simulink model "Update_E_Bike_model_without_controller"  (R2019b)
settings: Solver=VariableStepAuto  StartTime=0.0  StopTime=1000  RelTol=1e-3
InitFcn:
  | Rho_air= 1.225;
  | C_d=0.9;
  | A_d= 0.4;
  | Static_Friction_Coefficient =0.0015;
  | Dynamic_Friction_Coefficient= 0.0015;
  | Cyclist_weight=85;
  | Vehicle_mass = 5;
  | g = 9.81;
  | Wheel_Inertia = 0.45;
  | Bb=0.2;
  | Wheel_Radius = 0.3;
  | F_Rider = 100;
  | Brake_Pressure = 0;
  | Crank_Length = 0.150;
  | Angle_of_crank = [0:1:360;0:1:360;]';
  | Number_of_brake_pad = 2;
  | Coefficient_of_Brake_friction = 0.9;
  | Effective_Radius_of_Disc = 0.16;
  | Outer_Radius_of_Brake = 0.18;
  | Inner_Radius_of_Brake = 0.14;
  | Disc_Mass=0;
  | Heat_capacity=0;
  | Surface_Temp=0;
  | Ambient_Temp=0;
  | Thermal_Conductivity=1;
  | 
  | Motor_torque_constant = 1.41; % NM/A
  | Kb = (1/(190*2*pi/60)); %or  V/Wm (wm in rps) volt/rps
  | Jm =11.6 *10^-7; %kgm^2
  | Bm = ((Motor_torque_constant)*(20*10^-3)/(9080*2*pi/60));
  | Motor_resistance =250*10^-3; %ohm
  | L = .82*10^-3;% H(henry)
  | alpha_Conductor =0.0040;
  | Ref_Temp = 25;
  | Alpha_Magnet = -0.0020;
  | 
  | Current =2; %A
  | Internal_Resistance = 95*10^-3; %ohm
  | capacity = 14.5 ; %Ah
  | SOC_initial = 100;
  | Polarization_Resistance = 95*10^-3;
  | Polarization_Capacitance = 1*10^-7;
  | bp.SOC0_pct=00
undefined symbols (not defined in the file or in its folder): sigbuilder_block
(part 1 of 3)
settings Model: Creator=Avmash  LastModifiedBy=Avmash
settings DataIOCC: ReturnWorkspaceOutputs=off
settings DebuggingCC: AlgebraicLoopMsg=none  ArithmeticOperatorsInVariantConditions=warning
settings SFSimCC: SimUseLocalCustomCode=off  CustomCodeUndefinedFunction=UseInterfaceOnly
settings RTWCC: RTWUseLocalCustomCode=off

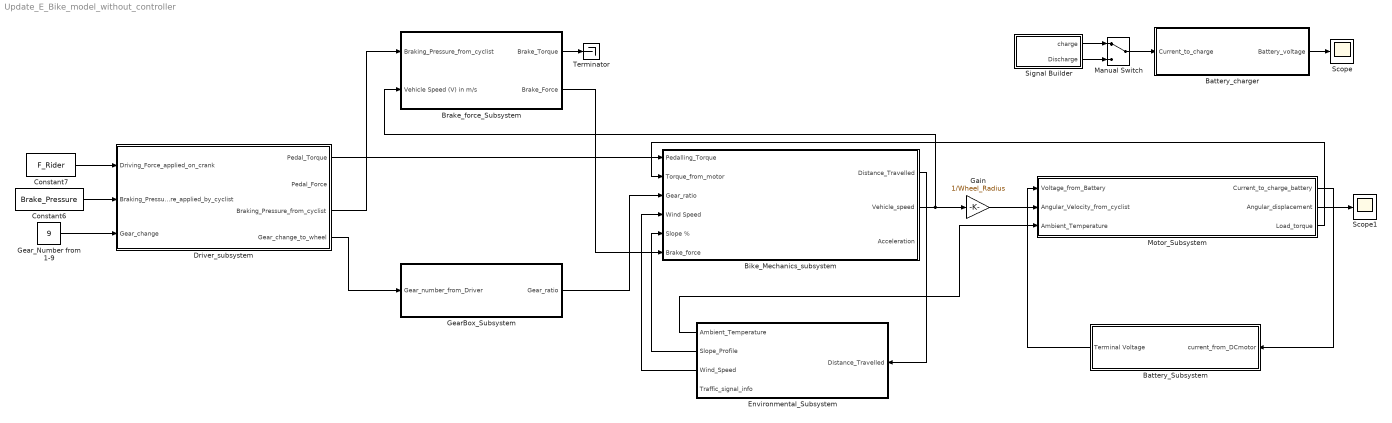
== system Update_E_Bike_model_without_controller ==
  Battery_Subsystem : Subsystem
  Battery_charger : Subsystem
  Bike_Mechanics_subsystem : Subsystem
  Brake_force_Subsystem : Subsystem
  Constant6 : Constant  Value=Brake_Pressure
  Constant7 : Constant  Value=F_Rider
  Driver_subsystem : Subsystem
  Environmental_Subsystem : Subsystem
  Gain : Gain  Gain=1/Wheel_Radius
  GearBox_Subsystem : Subsystem
  Gear_Number from 1-9 : Constant  Value=9
  Manual Switch : ManualSwitch
  Motor_Subsystem : Subsystem
  Scope : Scope
  Scope1 : Scope
  Signal Builder : Subsystem  Tag=STV Subsys  LoadFcn=sigbuilder_block('load');  StartFcn=sigbuilder_block('start');  StopFcn=sigbuilder_block('stop');  ClipboardFcn=sigbuilder_block('clipboard');  mask(Sigbuilder block){tuvar=[0:10]}
      mask help: Simulink:masks:SigbuilderBlock_MD
      mask init:
      | if ~strcmp(get_param(bdroot(gcbh),'SimulationStatus'),'stopped') tuvar = sigbuilder_block('maskInit'); end
      settings: CopyFcn=sigbuilder_block('copy');  DeleteFcn=sigbuilder_block('delete');  ModelCloseFcn=sigbuilder_block('modelClose');  PreSaveFcn=sigbuilder_block('preSave');  PauseFcn=sigbuilder_block('pause');  ContinueFcn=sigbuilder_block('continue');  NameChangeFcn=sigbuilder_block('namechange');  OpenFcn=sigbuilder_block('open',[6 30 1012.5 447.75 ]);  CloseFcn=sigbuilder_block('close');
      mask Display: plot(0, 0, 100, 100,[2, 2, 32, 32, 2], [68, 8, 8, 68, 68],[32, 2], [38, 38], [32, 19, 2],[53, 60, 44], [32, 17, 17, 2],[16, 16, 31, 31]);txt = getActiveGroup(gcbh);text(2, 100, txt,'verticalAlignment', 'top');
  Terminator : Terminator
  wires:
  Constant6/1 -> Driver_subsystem/2(Braking_Pressure_applied_by_cyclist)
  Gear_Number from 1-9/1 -> Driver_subsystem/3(Gear_change)
  Constant7/1 -> Driver_subsystem/1(Driving_Force_applied_on_crank)
  Brake_force_Subsystem/2(Brake_Force) -> Bike_Mechanics_subsystem/6("Brake_force ")
  Brake_force_Subsystem/1(Brake_Torque) -> Terminator/1
  Driver_subsystem/3(Braking_Pressure_from_cyclist) -> Brake_force_Subsystem/1(Braking_Pressure_from_cyclist)
  Driver_subsystem/1(Pedal_Torque) -> Bike_Mechanics_subsystem/1(Pedalling_Torque)
  Driver_subsystem/4(Gear_change_to_wheel) -> GearBox_Subsystem/1(Gear_number_from_Driver)
  GearBox_Subsystem/1(Gear_ratio) -> Bike_Mechanics_subsystem/3(Gear_ratio)
  Environmental_Subsystem/2(Slope_Profile) -> Bike_Mechanics_subsystem/5(Slope %)
  Environmental_Subsystem/3(Wind_Speed) -> Bike_Mechanics_subsystem/4(Wind Speed)
  Bike_Mechanics_subsystem/1(Distance_Travelled) -> Environmental_Subsystem/1(Distance_Travelled)
  Manual Switch/1 -> Battery_charger/1(Current_to_charge)
  Battery_charger/1(Battery_voltage) -> Scope/1
  Signal Builder/1(charge) -> Manual Switch/1
  Signal Builder/2(Discharge) -> Manual Switch/2
  Battery_Subsystem/1(Terminal Voltage) -> Motor_Subsystem/1(Voltage_from_Battery)
  Environmental_Subsystem/1(Ambient_Temperature) -> Motor_Subsystem/3(Ambient_Temperature)
  Motor_Subsystem/1(Current_to_charge_battery) -> Battery_Subsystem/1(current_from_DCmotor)
  Gain/1 -> Motor_Subsystem/2(Angular_Velocity_from_cyclist)
  Bike_Mechanics_subsystem/2(Vehicle_speed) -> Gain/1, Brake_force_Subsystem/2(Vehicle Speed (V) in m/s)
  Motor_Subsystem/3(Load_torque) -> Bike_Mechanics_subsystem/2(Torque_from_motor)
  Motor_Subsystem/2(Angular_displacement) -> Scope1/1

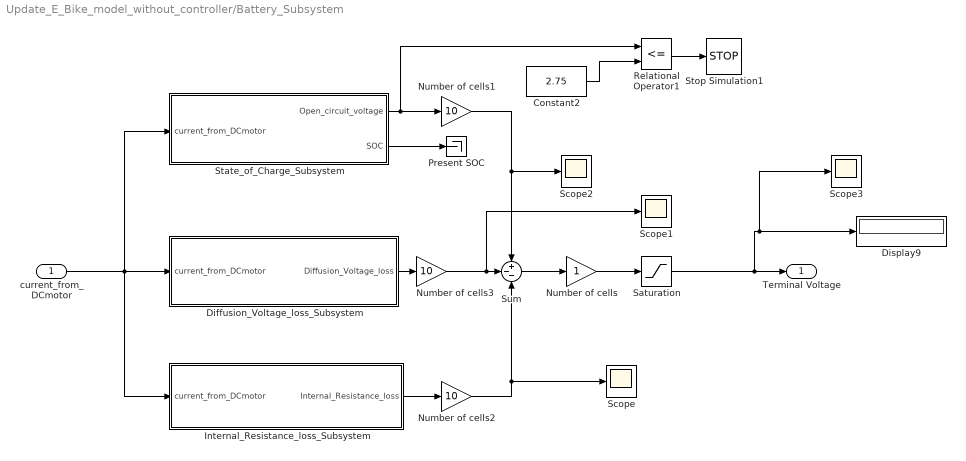
== system Update_E_Bike_model_without_controller/Battery_Subsystem ==
  current_from_DCmotor : Inport
  Constant2 : Constant  Value=2.75
  Diffusion_Voltage_loss_Subsystem : Subsystem
  Display9 : Display
  Internal_Resistance_loss_Subsystem : Subsystem
  Number of cells : Gain
  Number of cells1 : Gain  Gain=10
  Number of cells2 : Gain  Gain=10
  Number of cells3 : Gain  Gain=10
  Present SOC : Terminator
  Relational Operator1 : RelationalOperator  Operator=<=  OutDataTypeStr=boolean  RndMeth=Simplest
  Saturation : Saturate  UpperLimit=inf  LowerLimit=0
  Scope{,1..3} (4 alike) : Scope
  "State_of_Charge_Subsystem " : Subsystem
  Stop Simulation1 : Stop
  Sum : Sum  Inputs=+--
  Terminal Voltage : Outport  VectorParamsAs1DForOutWhenUnconnected=off
  wires:
  current_from_DCmotor/1 -> Internal_Resistance_loss_Subsystem/1(current_from_DCmotor), "State_of_Charge_Subsystem "/1(current_from_DCmotor), Diffusion_Voltage_loss_Subsystem/1(current_from_DCmotor)
  Sum/1 -> Number of cells/1
  "State_of_Charge_Subsystem "/2(SOC) -> Present SOC/1
  Internal_Resistance_loss_Subsystem/1(Internal_Resistance_loss) -> Number of cells2/1
  Number of cells/1 -> Saturation/1
  Diffusion_Voltage_loss_Subsystem/1(Diffusion_Voltage_loss) -> Number of cells3/1
  Saturation/1 -> Terminal Voltage/1, Scope3/1, Display9/1
  Relational Operator1/1 -> Stop Simulation1/1
  Constant2/1 -> Relational Operator1/2
  "State_of_Charge_Subsystem "/1(Open_circuit_voltage) -> Number of cells1/1, Relational Operator1/1
  Number of cells2/1 -> Scope/1, Sum/3
  Number of cells3/1 -> Scope1/1, Sum/2
  Number of cells1/1 -> Scope2/1, Sum/1

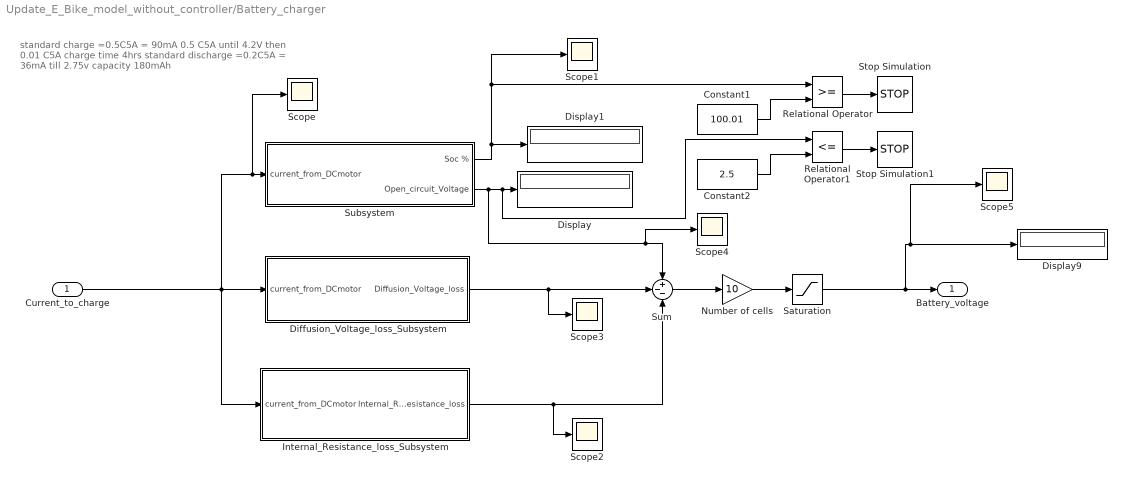
== system Update_E_Bike_model_without_controller/Battery_charger ==
  note: standard charge =0.5C5A = 90mA
      | 0.5 C5A until 4.2V then 0.01 C5A charge time 4hrs
      |
      | standard discharge =0.2C5A = 36mA till 2.75v
      |
      | capacity 180mAh
  Current_to_charge : Inport
  Constant1 : Constant  Value=100.01
  Constant2 : Constant  Value=2.5
  Diffusion_Voltage_loss_Subsystem : Subsystem
  Display : Display
  Display1 : Display
  Display9 : Display
  Internal_Resistance_loss_Subsystem : Subsystem
  Number of cells : Gain  Gain=10
  Relational Operator : RelationalOperator  OutDataTypeStr=boolean  RndMeth=Simplest
  Relational Operator1 : RelationalOperator  Operator=<=  OutDataTypeStr=boolean  RndMeth=Simplest
  Saturation : Saturate  UpperLimit=inf  LowerLimit=0
  Scope{,1..5} (6 alike) : Scope
  Stop Simulation : Stop
  Stop Simulation1 : Stop
  Subsystem : Subsystem
  Sum : Sum  Inputs=+--
  Battery_voltage : Outport  VectorParamsAs1DForOutWhenUnconnected=off
  wires:
  Saturation/1 -> Battery_voltage/1, Scope5/1, Display9/1
  Constant2/1 -> Relational Operator1/2
  Subsystem/2(Open_circuit_Voltage) -> Relational Operator1/1, Display/1, Scope4/1, Sum/1
  Diffusion_Voltage_loss_Subsystem/1(Diffusion_Voltage_loss) -> Sum/2, Scope3/1
  Current_to_charge/1 -> Scope/1, Subsystem/1(current_from_DCmotor), Internal_Resistance_loss_Subsystem/1(current_from_DCmotor), Diffusion_Voltage_loss_Subsystem/1(current_from_DCmotor)
  Sum/1 -> Number of cells/1
  Subsystem/1(Soc %) -> Relational Operator/1, Scope1/1, Display1/1
  Internal_Resistance_loss_Subsystem/1(Internal_Resistance_loss) -> Sum/3, Scope2/1
  Number of cells/1 -> Saturation/1
  Relational Operator/1 -> Stop Simulation/1
  Constant1/1 -> Relational Operator/2
  Relational Operator1/1 -> Stop Simulation1/1

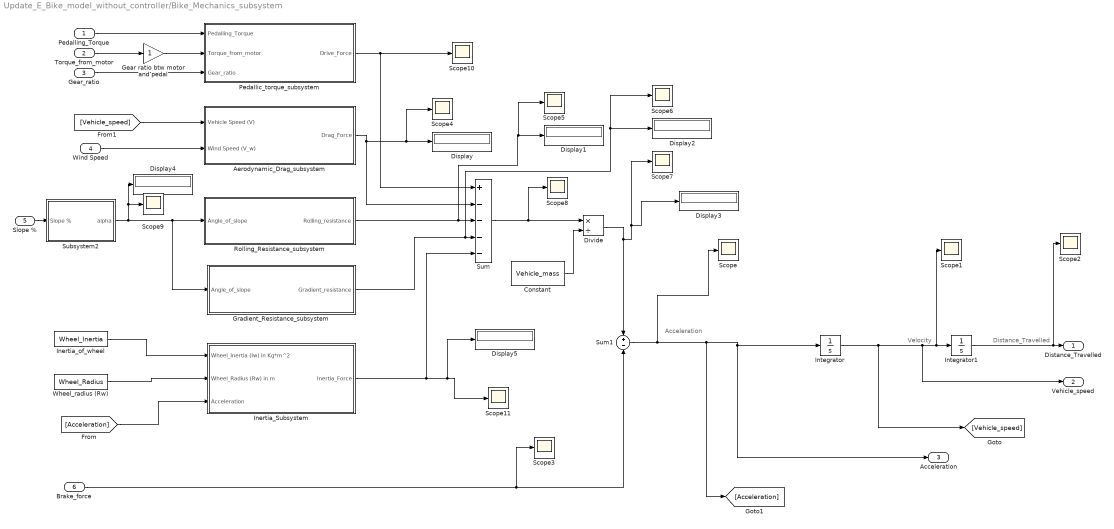
== system Update_E_Bike_model_without_controller/Bike_Mechanics_subsystem ==
  note: Acceleration
  note: Velocity
  note: Distance_Travelled
  Pedalling_Torque : Inport
  Torque_from_motor : Inport  Port=2
  Gear_ratio : Inport  Port=3
  Wind Speed : Inport  Port=4
  Slope % : Inport  Port=5
  "Brake_force " : Inport  Port=6
  Aerodynamic_Drag_subsystem : Subsystem
  Constant : Constant  Value=Vehicle_mass
  Display{,1..5} (6 alike) : Display
  Divide : Product  Inputs=*/
  Gear ratio btw motor and pedal : Gain
  Gradient_Resistance_subsystem : Subsystem
  Inertia_Subsystem : Subsystem
  Inertia_of_wheel : Constant  Value=Wheel_Inertia
  Integrator : Integrator
  Integrator1 : Integrator
  Pedallic_torque_subsystem : Subsystem
  Rolling_Resistance_subsystem : Subsystem
  Scope{,1..11} (12 alike) : Scope
  Subsystem2 : Subsystem
  Sum : Sum  Inputs=+----
  Sum1 : Sum  Inputs=+-
  "Wheel_radius (Rw) " : Constant  Value=Wheel_Radius
  Distance_Travelled : Outport  VectorParamsAs1DForOutWhenUnconnected=off
  Vehicle_speed : Outport  Port=2  VectorParamsAs1DForOutWhenUnconnected=off
  Acceleration : Outport  Port=3  VectorParamsAs1DForOutWhenUnconnected=off
  wires:
  Inertia_Subsystem/1(Inertia_Force) -> Sum/5, Display5/1, Scope11/1
  [Acceleration] -> Inertia_Subsystem/3(Acceleration)
  Rolling_Resistance_subsystem/1(Rolling_resistance) -> Sum/3, Scope5/1, Display1/1
  "Wheel_radius (Rw) "/1 -> Inertia_Subsystem/2(Wheel_Radius (Rw) in m)
  Gear ratio btw motor and pedal/1 -> Pedallic_torque_subsystem/2(Torque_from_motor)
  [Vehicle_speed] -> Aerodynamic_Drag_subsystem/1(Vehicle Speed (V))
  Pedallic_torque_subsystem/1(Drive_Force) -> Sum/1, Scope10/1
  Gradient_Resistance_subsystem/1(Gradient_resistance) -> Scope6/1, Display2/1, Sum/4
  Wind Speed/1 -> Aerodynamic_Drag_subsystem/2("Wind Speed (V_w) ")
  Aerodynamic_Drag_subsystem/1("Drag_Force ") -> Sum/2, Scope4/1, Display/1
  Inertia_of_wheel/1 -> Inertia_Subsystem/1(Wheel_Inertia (Iw) in Kg*m^2)
  Constant/1 -> Divide/2
  Sum1/1 -> [Acceleration], Acceleration/1, Integrator/1, Scope/1
  Integrator/1 -> [Vehicle_speed], Scope1/1, Integrator1/1, Vehicle_speed/1
  Divide/1 -> Display3/1, Scope7/1, Sum1/1
  Subsystem2/1(alpha) -> Display4/1, Scope9/1, Gradient_Resistance_subsystem/1(Angle_of_slope), Rolling_Resistance_subsystem/1(Angle_of_slope)
  Torque_from_motor/1 -> Gear ratio btw motor and pedal/1
  Sum/1 -> Scope8/1, Divide/1
  Gear_ratio/1 -> Pedallic_torque_subsystem/3(Gear_ratio)
  "Brake_force "/1 -> Scope3/1, Sum1/2
  Pedalling_Torque/1 -> Pedallic_torque_subsystem/1(Pedalling_Torque)
  Integrator1/1 -> Scope2/1, Distance_Travelled/1
  Slope %/1 -> Subsystem2/1(Slope %)

== system Update_E_Bike_model_without_controller/Brake_force_Subsystem ==
  Braking_Pressure_from_cyclist : Inport
  Vehicle Speed (V) in m/s : Inport  Port=2
  Brake_Distance_Subsystem : Subsystem
  Brake_subsystem : Subsystem
  Display : Display
  Display1 : Display
  Inner_Radius_of_Brake_pad : Constant  Value=Inner_Radius_of_Brake
  Outer_Radius_of_Brake_pad : Constant  Value=Outer_Radius_of_Brake
  Thermal_Gradient_Subsystem : Subsystem
  Brake_Torque : Outport
  Brake_Force : Outport  Port=2
  wires:
  Brake_subsystem/2(Brake_force) -> Brake_Force/1, Brake_Distance_Subsystem/1(Brake_Force)
  Braking_Pressure_from_cyclist/1 -> Brake_subsystem/1(Max_Pressure_applied_on_brake_lever)
  Vehicle Speed (V) in m/s/1 -> Brake_Distance_Subsystem/2(Vehicle_speed)
  Outer_Radius_of_Brake_pad/1 -> Brake_subsystem/2(Outer_Radius_of_Brake_pad), Thermal_Gradient_Subsystem/1(Outer_Radius_of_Brake_pad)
  Inner_Radius_of_Brake_pad/1 -> Thermal_Gradient_Subsystem/2(Inner_Radius_of_Brake_pad), Brake_subsystem/3(Inner_Radius_of_Brake_pad)
  Thermal_Gradient_Subsystem/1(Thermal_Gradient) -> Display1/1
  Brake_subsystem/1(Brake_Torque) -> Brake_Torque/1
  Brake_Distance_Subsystem/1(Brake_Distance) -> Display/1

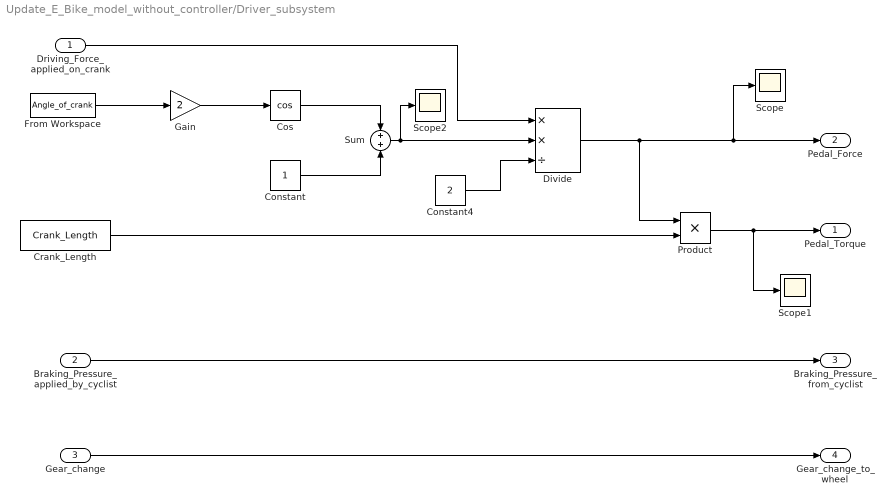
== system Update_E_Bike_model_without_controller/Driver_subsystem ==
  Driving_Force_applied_on_crank : Inport
  Braking_Pressure_applied_by_cyclist : Inport  Port=2
  Gear_change : Inport  Port=3
  Constant : Constant
  Constant4 : Constant  Value=2
  Cos : Trigonometry  Operator=cos
  Crank_Length : Constant  Value=Crank_Length
  Divide : Product  Inputs=**/
  From Workspace : FromWorkspace  VariableName=Angle_of_crank  SampleTime=0
  Gain : Gain  Gain=2
  Product : Product
  Scope : Scope
  Scope1 : Scope
  Scope2 : Scope
  Sum : Sum
  Pedal_Torque : Outport
  Pedal_Force : Outport  Port=2
  Braking_Pressure_from_cyclist : Outport  Port=3
  Gear_change_to_wheel : Outport  Port=4  VectorParamsAs1DForOutWhenUnconnected=off
  wires:
  Divide/1 -> Scope/1, Pedal_Force/1, Product/1
  Gain/1 -> Cos/1
  Constant/1 -> Sum/2
  Cos/1 -> Sum/1
  Product/1 -> Scope1/1, Pedal_Torque/1
  Constant4/1 -> Divide/3
  Driving_Force_applied_on_crank/1 -> Divide/1
  Sum/1 -> Scope2/1, Divide/2
  Crank_Length/1 -> Product/2
  Braking_Pressure_applied_by_cyclist/1 -> Braking_Pressure_from_cyclist/1
  From Workspace/1 -> Gain/1
  Gear_change/1 -> Gear_change_to_wheel/1

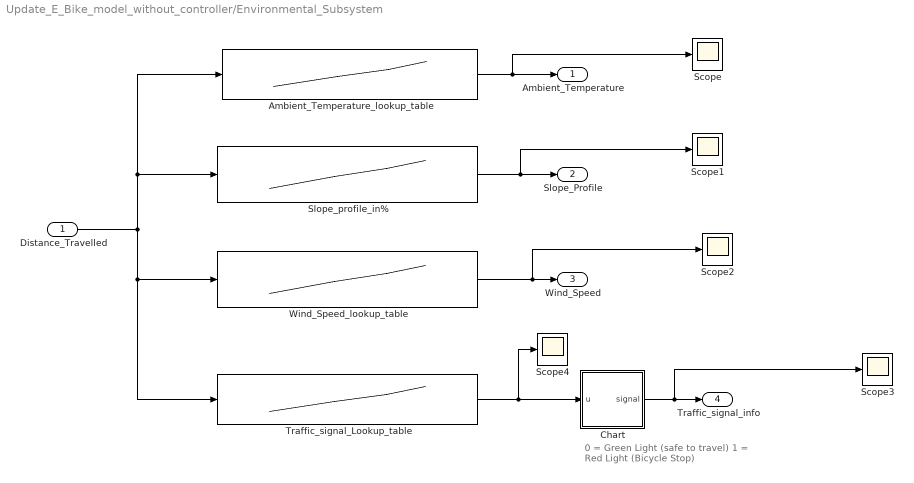
== system Update_E_Bike_model_without_controller/Environmental_Subsystem ==
  note: 0 = Green Light (safe to travel)
      | 1 = Red Light (Bicycle Stop)
  Distance_Travelled : Inport
  Ambient_Temperature_lookup_table : Lookup_n-D  NumberOfTableDimensions=1  BreakpointsForDimension1=[0 12000]  Table=[25 25]  InternalRulePriority=Speed  RndMeth=Simplest  InputSameDT=on
  Chart : Stateflow chart  BlockKeywords=__PRM__SERIALIZED__DATA__:Stateflow Chart,Stateflow Diagram  TreatAsAtomicUnit=on
  Scope{,1..4} (5 alike) : Scope
  Slope_profile_in% : Lookup_n-D  NumberOfTableDimensions=1  BreakpointsForDimension1=|  Table=|  InternalRulePriority=Speed  RndMeth=Simplest  InputSameDT=on
      BreakpointsForDimension1=|
      | [0000,
      | 0015,
      | 0056,
      | 0099,
      | 0108,
      | 0118,
      | 0132,
      | 0142,
      | 0160,
      | 0170,
      | 0186,
      | 0228,
      | 0293,
      | 0336,
      | 0363,
      | 0381,
      | 0391,
      | 0402,
      | 0437,
      | 0478,
      | 0538,
      | 0565,
      | 0582,
      | 0591,
      | 0611,
      | 0640,
      | 0675,
      | 0684,
      | 0699,
      | 0757,
      | 0777,
      | 0788,
      | 0820,
      | 0823,
      | 0837,
      | 0841,
      | 0863,
      | 0880,
      | 0900,
      | 0918,
      | 0948,
      | 0985,
      | 1016,
      | 1037,
      | 1051,
      | 1061,
      | 1082,
      | 1113,
      | 1134,
      | 1142,
      | 1151,
      | 1165,
      | 1176,
      | 1187,
      | 1200,
      | 1216,
      | 1234,
      | 1277,
      | 1341,
      | 1373,
      | 1401,
      | 1452,
      | 1486,
      | 1497,
      | 1507,
      | 1520,
      | 1528,
      | 1557,
      | 1649,
      | 1694,
      | 1716,
      | 1767,
      | 1827,
      | 1898,
      | 1946,
      | 2017,
      | 2030,
      | 2040,
      | 2056,
      | 2110,
      | 2201,
      | 2231,
      | 2242,
      | 2325,
      | 2412,
      | 2504,
      | 2530,
      | 2570,
      | 2607,
      | 2640,
      | 2665,
      | 2713,
      | 2730,
      | 2752,
      | 2763,
      | 2774,
      | 2863,
      | 2961,
      | 3095,
      | 3167,
      | 3268,
      | 3368,
      | 3384,
      | 3418,
      | 3480,
      | 3503,
      | 3562,
      | 3601,
      | 3635,
      | 3719,
      | 3748,
      | 3768,
      | 3844,
      | 3916,
      | 4078,
      | 4224,
      | 4305,
      | 4357,
      | 4398,
      | 4445,
      | 4493,
      | 4548,
      | 4641,
      | 4770,
      | 4916,
      | 5015,
      | 5084,
      | 5110,
      | 5212,
      | 5458,
      | 5491,
      | 5525,
      | 5541,
      | 5551,
      | 5562,
      | 5574,
      | 5591,
      | 5622,
      | 5652,
      | 5665,
      | 5727,
      | 5806,
      | 5856,
      | 5914,
      | 5974,
      | 6031,
      | 6097,
      | 6322,
      | 6482,
      | 6528,
      | 6632,
      | 6688,
      | 6763,
      | 6810,
      | 6853,
      | 6910,
      | 6951,
      | 6998,
      | 7051,
      | 7185,
      | 7248,
      | 7303,
      | 7349,
      | 7386,
      | 7421,
      | 7455,
      | 7492,
      | 7530,
      | 7567,
      | 7609,
      | 7691,
      | 7747,
      | 7751,
      | 7764,
      | 7775,
      | 7808,
      | 7833,
      | 8143,
      | 8170,
      | 8180,
      | 8210,
      | 8811,
      | 8980,
      | 9047,
      | 9065,
      | 9086,
      | 9104,
      | 9141,
      | 9168,
      | 9191,
      | 9215,
      | 9249,
      | 9296,
      | 9348,
      | 9405,
      | 9426,
      | 9442,
      | 9473,
      | 9515,
      | 9550,
      | 9581,
      | 9601,
      | 9627,
      | 9652,
      | 9682,
      | 9735,
      | 9760,
      | 9774,
      | 9784,
      | 9797,
      | 9818,
      | 9838,
      | 9858,
      | 9880,
      | 9972,
      | 10015,
      | 10110,
      | 10128,
      | 10180,
      | 10196,
      | 10262,
      | 10271,
      | 10295,
      | 10311,
      | 10379,
      | 10402,
      | 10421,
      | 10433,
      | 10449,
      | 10470,
      | 10483,
      | 10492,
      | 10501,
      | 10541,
      | 10561,
      | 10573,
      | 10601,
      | 10626,
      | 10652,
      | 10709,
      | 10748,
      | 10809,
      | 10840,
      | 10860,
      | 10877,
      | 10888,
      | 10897,
      | 10912,
      | 10927,
      | 10988,
      | 11013,
      | 11027,
      | 11042,
      | 11084,
      | 11094,
      | 11117,
      | 11138,
      | 11167,
      | 11197,
      | 11251,
      | 11270,
      | 11290,
      | 11304,
      | 11320,
      | 11335,
      | 11351,
      | 11367,
      | 11446,
      | 11492,
      | 11514,
      | 11529,
      | 11540,
      | 11579,
      | 11596,
      | 11645,
      | 11667,
      | 11674,
      | 11689,
      | 11702,
      | 11800
      | ]
      Table=|
      | [0,
      | 0.487804878,
      | 0.23255814,
      | 0,
      | 1,
      | 0,
      | 0,
      | 0,
      | 0,
      | 0,
      | 0.714285714,
      | 0.769230769,
      | 0.697674419,
      | 0.740740741,
      | 0,
      | 0,
      | 0,
      | 0.285714286,
      | 0.243902439,
      | 0.166666667,
      | 0.37037037,
      | 0.588235294,
      | 0,
      | 0,
      | 0,
      | 0,
      | 0,
      | 0,
      | 0.344827586,
      | 0,
      | 0,
      | 0.3125,
      | 0,
      | 0.714285714,
      | 0,
      | 0,
      | 0,
      | 0,
      | 0,
      | 0.333333333,
      | 0.27027027,
      | 0,
      | 0,
      | 0,
      | 1,
      | 0,
      | 0,
      | 0,
      | 0,
      | 0,
      | 0,
      | 0,
      | 0,
      | 0,
      | 0,
      | 0,
      | 0,
      | 0,
      | 0.3125,
      | 0,
      | 0,
      | 0,
      | 0,
      | 0,
      | 0,
      | 0,
      | 0.344827586,
      | 0,
      | 0,
      | 0,
      | 0,
      | 0,
      | 0,
      | 0,
      | 0,
      | 0,
      | 0,
      | 0,
      | 0.185185185,
      | 0,
      | 0,
      | 0,
      | 0,
      | 0,
      | 0,
      | 0,
      | 0,
      | 0,
      | 0,
      | 0,
      | 0,
      | 0.588235294,
      | 0,
      | 0,
      | 0,
      | 0.112359551,
      | 0,
      | 0,
      | 0,
      | 0,
      | 0.1,
      | 0,
      | 0,
      | 0,
      | 0.434782609,
      | 0.169491525,
      | 0,
      | 0,
      | 0,
      | 0,
      | 0,
      | 0,
      | 0,
      | 0.061728395,
      | 0,
      | 0,
      | 0,
      | 0,
      | 0,
      | 0,
      | 0,
      | 0,
      | 0,
      | 0,
      | 0,
      | 0,
      | 0,
      | 0,
      | 0,
      | 0.303030303,
      | 0,
      | 0.625,
      | 0,
      | 0,
      | 0.833333333,
      | 0,
      | 0.322580645,
      | 0,
      | 0,
      | 0.322580645,
      | 0.379746835,
      | 0,
      | 0,
      | 0,
      | 0.175438596,
      | 0,
      | 0,
      | 0,
      | 0,
      | 0.096153846,
      | 0,
      | 0.133333333,
      | 0.212765957,
      | 0,
      | 0,
      | 0,
      | 0.212765957,
      | 0,
      | 0,
      | 0,
      | 0,
      | 0.217391304,
      | 0,
      | 0,
      | 0,
      | 0,
      | 0,
      | 0,
      | 0.238095238,
      | 0.12195122,
      | 0.357142857,
      | 0,
      | 0,
      | 0,
      | 0,
      | 0.4,
      | 0,
      | 0,
      | 0,
      | 0.333333333,
      | 0,
      | 0,
      | 0.149253731,
      | 0,
      | 0,
      | 0,
      | 0,
      | 0.37037037,
      | 0,
      | 0.416666667,
      | 0,
      | 0.212765957,
      | 0.192307692,
      | 0.175438596,
      | 0,
      | 0,
      | 0,
      | 0.238095238,
      | 0.285714286,
      | 0,
      | 0.5,
      | 0.384615385,
      | 0.4,
      | 0,
      | 0,
      | 0,
      | 0,
      | 0,
      | 0,
      | 0,
      | 0,
      | 0,
      | 0,
      | 0,
      | 0,
      | 0,
      | 0,
      | 0.192307692,
      | 0,
      | 0,
      | 0,
      | 0,
      | 0,
      | 0,
      | 0,
      | 0,
      | 0,
      | 0,
      | 0,
      | 0,
      | 0,
      | 0,
      | 0,
      | 0.5,
      | 0,
      | 0,
      | 0,
      | 0,
      | 0,
      | 0,
      | 0,
      | 0,
      | 0,
      | 0.588235294,
      | 0,
      | 0,
      | 0,
      | 0,
      | 0,
      | 0,
      | 0,
      | 0,
      | 0,
      | 0,
      | 0,
      | 0,
      | 0,
      | 0,
      | 0,
      | 0,
      | 0,
      | 0,
      | 0.625,
      | 0,
      | 0,
      | 0,
      | 0.126582278,
      | 0,
      | 0,
      | 0,
      | 0,
      | 0,
      | 0,
      | 0,
      | 0,
      | 0,
      | 0,
      | 0,
      | 0,
      | 0
      | ]
  Traffic_signal_Lookup_table : Lookup_n-D  NumberOfTableDimensions=1  BreakpointsForDimension1=|  Table=|  InternalRulePriority=Speed  RndMeth=Simplest  InputSameDT=on
      BreakpointsForDimension1=|
      | [0,
      | 1352.604,
      | 1352.624,
      | 1352.644,
      | 2594.125,
      | 2594.145,
      | 2594.165,
      | 5283.812,
      | 5283.832,
      | 5283.852,
      | 7423.782,
      | 7423.802,
      | 7423.822,
      | 9090.133,
      | 9090.153,
      | 9090.173,
      | 9442.834,
      | 9442.854,
      | 9442.874,
      | 9911.784,
      | 9911.804,
      | 9911.824,
      | 10337.11,
      | 10337.31,
      | 10337.51,
      | 10698.74,
      | 10698.94,
      | 10699.14,
      | 11070.92,
      | 11071.12,
      | 11071.32,
      | 11082.84,
      | 11083.04,
      | 11083.24,
      | 11800
      | ]
      Table=|
      | [
      | 0,
      | 0,
      | 1,
      | 0,
      | 0,
      | 1,
      | 0,
      | 0,
      | 1,
      | 0,
      | 0,
      | 1,
      | 0,
      | 0,
      | 1,
      | 0,
      | 0,
      | 1,
      | 0,
      | 0,
      | 1,
      | 0,
      | 0,
      | 1,
      | 0,
      | 0,
      | 1,
      | 0,
      | 0,
      | 1,
      | 0,
      | 0,
      | 1,
      | 0,
      | 0]
  Wind_Speed_lookup_table : Lookup_n-D  NumberOfTableDimensions=1  BreakpointsForDimension1=[0 12000]  Table=[0 0]  InternalRulePriority=Speed  RndMeth=Simplest  InputSameDT=on
  Ambient_Temperature : Outport  VectorParamsAs1DForOutWhenUnconnected=off
  Slope_Profile : Outport  Port=2  VectorParamsAs1DForOutWhenUnconnected=off
  Wind_Speed : Outport  Port=3  VectorParamsAs1DForOutWhenUnconnected=off
  Traffic_signal_info : Outport  Port=4  VectorParamsAs1DForOutWhenUnconnected=off
  wires:
  Distance_Travelled/1 -> Wind_Speed_lookup_table/1, Traffic_signal_Lookup_table/1, Slope_profile_in%/1, Ambient_Temperature_lookup_table/1
  Wind_Speed_lookup_table/1 -> Scope2/1, Wind_Speed/1
  Ambient_Temperature_lookup_table/1 -> Ambient_Temperature/1, Scope/1
  Slope_profile_in%/1 -> Slope_Profile/1, Scope1/1
  Chart/1(signal) -> Scope3/1, Traffic_signal_info/1
  Traffic_signal_Lookup_table/1 -> Scope4/1, Chart/1(u)

== system Update_E_Bike_model_without_controller/GearBox_Subsystem ==
  Gear_number_from_Driver : Inport
  Crankset_Teeth : Constant  Value=34
  Divide : Product  Inputs=*/
  Gear_Box_Subsystem : Subsystem
  Gear_ratio : Outport  VectorParamsAs1DForOutWhenUnconnected=off
  wires:
  Divide/1 -> Gear_ratio/1
  Gear_number_from_Driver/1 -> Gear_Box_Subsystem/1(Gear_Number)
  Gear_Box_Subsystem/1(Final_Gear_Teeth) -> Divide/1
  Crankset_Teeth/1 -> Divide/2

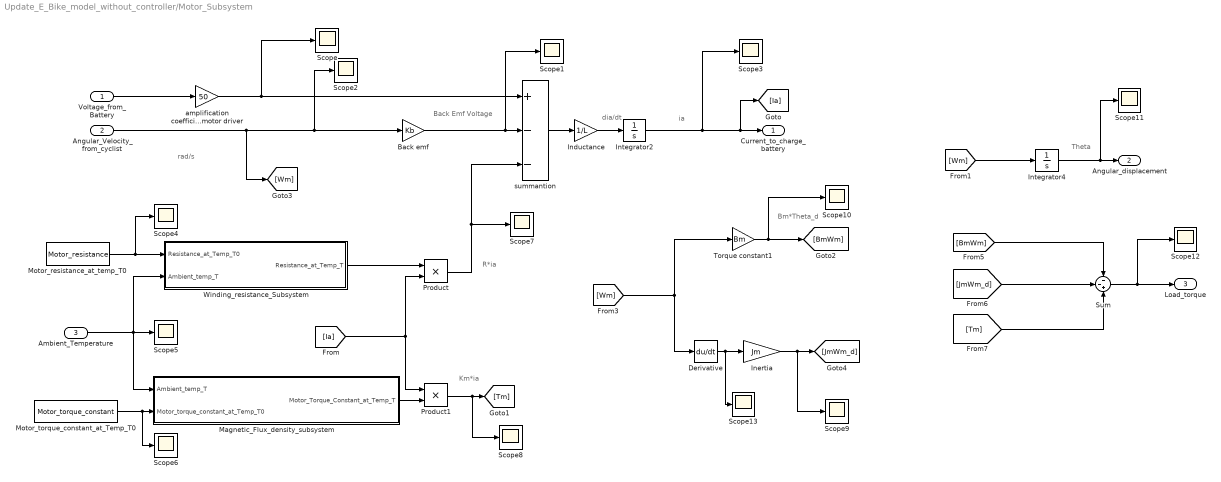
== system Update_E_Bike_model_without_controller/Motor_Subsystem ==
  note: ia
  note: dia/dt
  note: rad/s
  note: R*ia
  note: Km*ia
  note: Theta
  note: Bm*Theta_d
  note: Back Emf Voltage
  Voltage_from_Battery : Inport
  Angular_Velocity_from_cyclist : Inport  Port=2
  Ambient_Temperature : Inport  Port=3
  " amplification coefficient of the motor driver" : Gain  Gain=50
  Back emf : Gain  Gain=Kb
  Derivative : Derivative
  Inductance : Gain  Gain=1/L
  Inertia : Gain  Gain=Jm
  Integrator2 : Integrator
  Integrator4 : Integrator
  Magnetic_Flux_density_subsystem : Subsystem
  Motor_resistance_at_temp_T0 : Constant  Value=Motor_resistance  SampleTime=-1
  Motor_torque_constant_at_Temp_T0 : Constant  Value=Motor_torque_constant  SampleTime=-1
  Product : Product
  Product1 : Product
  Scope{,1..13} (14 alike) : Scope
  Sum : Sum  Inputs=--+
  Torque constant1 : Gain  Gain=Bm
  Winding_resistance_Subsystem : Subsystem
  summantion : Sum  Inputs=+--
  Current_to_charge_battery : Outport  VectorParamsAs1DForOutWhenUnconnected=off
  Angular_displacement : Outport  Port=2  VectorParamsAs1DForOutWhenUnconnected=off
  Load_torque : Outport  Port=3
  wires:
  Voltage_from_Battery/1 -> " amplification coefficient of the motor driver"/1
  Back emf/1 -> Scope1/1, summantion/2
  Inductance/1 -> Integrator2/1
  summantion/1 -> Inductance/1
  [Wm] -> Integrator4/1
  Motor_resistance_at_temp_T0/1 -> Scope4/1, Winding_resistance_Subsystem/1(Resistance_at_Temp_T0)
  Product/1 -> summantion/3, Scope7/1
  Ambient_Temperature/1 -> Winding_resistance_Subsystem/2(Ambient_temp_T), Scope5/1, Magnetic_Flux_density_subsystem/1(Ambient_temp_T)
  Motor_torque_constant_at_Temp_T0/1 -> Scope6/1, Magnetic_Flux_density_subsystem/2(Motor_torque_constant_at_Temp_T0)
  [Ia] -> Product1/1, Product/2
  Magnetic_Flux_density_subsystem/1(Motor_Torque_Constant_at_Temp_T) -> Product1/2
  Torque constant1/1 -> Scope10/1, [BmWm]
  Product1/1 -> Scope8/1, [Tm]
  Integrator4/1 -> Scope11/1, Angular_displacement/1
  Winding_resistance_Subsystem/1(Resistance_at_Temp_T) -> Product/1
  Angular_Velocity_from_cyclist/1 -> [Wm], Scope2/1, Back emf/1
  [Wm] -> Torque constant1/1, Derivative/1
  Derivative/1 -> Scope13/1, Inertia/1
  Inertia/1 -> Scope9/1, [JmWm_d]
  Sum/1 -> Scope12/1, Load_torque/1
  [Tm] -> Sum/3
  [JmWm_d] -> Sum/2
  [BmWm] -> Sum/1
  Integrator2/1 -> Scope3/1, [Ia], Current_to_charge_battery/1
  " amplification coefficient of the motor driver"/1 -> Scope/1, summantion/1

== system Update_E_Bike_model_without_controller/Signal Builder ==
  Demux : Demux  Tag=STV Demux  Outputs=2
  FromWs : FromWorkspace  Tag=STV FromWs  VariableName=tuvar  SampleTime=0
      SigBuilderData=|
      | common.afterFinalStr = 'Extrapolate'
      | common.sampleTime = 0
      | dataSet.timeRange = [0 14400]
      | dataSet.name = 'Group 1'
      | sbobj.Groups.Name = 'Group 1'
      | sbobj.Groups.Signals(1).Name = 'charge'
      | sbobj.Groups.Signals(1).XData = [0 6950 7150 14400]
      | sbobj.Groups.Signals(1).YData = [0.09 0.09 0.0018 0.0018]
      | sbobj.Groups.Signals(2).Name = 'Discharge'
      | sbobj.Groups.Signals(2).XData = [0 14400]
      | sbobj.Groups.Signals(2).YData = [-0.036 -0.036]
      | sbobj.Groups.TimeRange = [0 14400]
  charge : Outport  Tag=STV Outport
  Discharge : Outport  Tag=STV Outport  Port=2
  wires:
  FromWs/1 -> Demux/1
  Demux/1 -> charge/1
  Demux/2 -> Discharge/1

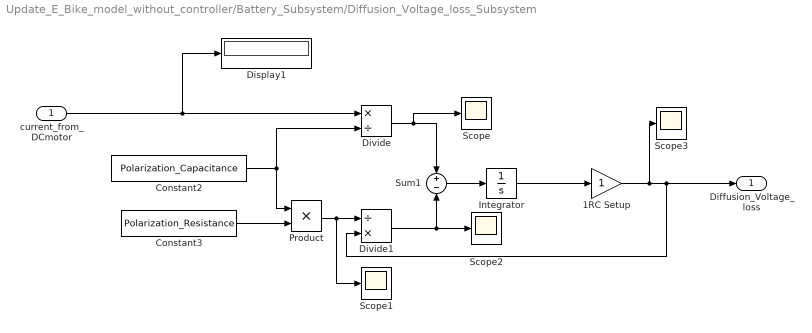
== system Update_E_Bike_model_without_controller/Battery_Subsystem/Diffusion_Voltage_loss_Subsystem ==
  current_from_DCmotor : Inport
  1RC Setup : Gain
  Constant2 : Constant  Value=Polarization_Capacitance  SampleTime=-1
  Constant3 : Constant  Value=Polarization_Resistance  SampleTime=-1
  Display1 : Display
  Divide : Product  Inputs=*/
  Divide1 : Product  Inputs=/*
  Integrator : Integrator
  Product : Product
  Scope{,1..3} (4 alike) : Scope
  Sum1 : Sum  Inputs=+|-
  Diffusion_Voltage_loss : Outport  VectorParamsAs1DForOutWhenUnconnected=off
  wires:
  Divide/1 -> Scope/1, Sum1/1
  Integrator/1 -> 1RC Setup/1
  Divide1/1 -> Sum1/2, Scope2/1
  Constant3/1 -> Product/2
  Product/1 -> Scope1/1, Divide1/1
  Sum1/1 -> Integrator/1
  current_from_DCmotor/1 -> Display1/1, Divide/1
  Constant2/1 -> Product/1, Divide/2
  1RC Setup/1 -> Scope3/1, Divide1/2, Diffusion_Voltage_loss/1

== system Update_E_Bike_model_without_controller/Battery_Subsystem/Internal_Resistance_loss_Subsystem ==
  current_from_DCmotor : Inport
  Constant : Constant  Value=Internal_Resistance  SampleTime=-1
  Product1 : Product
  Internal_Resistance_loss : Outport  VectorParamsAs1DForOutWhenUnconnected=off
  wires:
  current_from_DCmotor/1 -> Product1/1
  Constant/1 -> Product1/2
  Product1/1 -> Internal_Resistance_loss/1
